simulink model "ex5"  (R2025b)
settings: Solver=VariableStepAuto  StartTime=0.0  StopTime=10.0  RelTol=1e-3
settings Model: Creator=vladl  LastModifiedBy=vladl

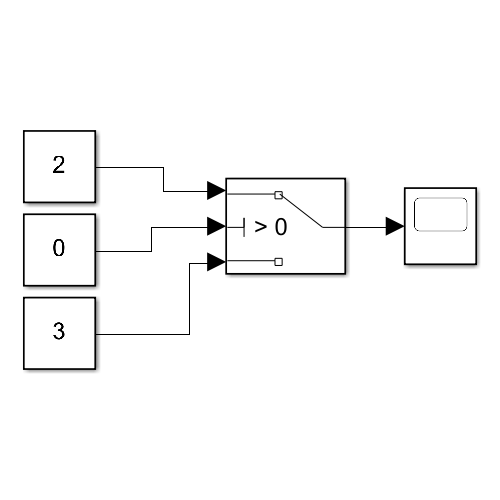
[thumbnail: Simulink's stored preview of the top-level diagram]
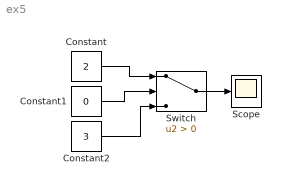
== system ex5 ==
  Constant : Constant  Value=2
  Constant1 : Constant  Value=0
  Constant2 : Constant  Value=3
  Scope : Scope
      settings: ActiveDisplayYMinimum=2  ActiveDisplayYMaximum=4
  Switch : Switch  Criteria=u2 > Threshold  SaturateOnIntegerOverflow=off  InputSameDT=off
  wires:
  Constant1/1 -> Switch/2
  Constant/1 -> Switch/1
  Constant2/1 -> Switch/3
  Switch/1 -> Scope/1
